simulink model "uas_hoops"  (R2021a)
settings: Solver=FixedStepAuto  StartTime=0.0  StopTime=1  FixedStep=0.04  RelTol=1e-3
model workspace: external: MAT-File (data not in the file)
libraries: robotlib x4
settings Model: EnablePacing=on  OrderedModelArguments=off  Creator=david  LastModifiedBy=david
settings SolverCC: AlgebraicLoopSolver=TrustRegion
settings DataIOCC: LimitDataPoints=on  MaxDataPoints=10000
settings OptimizationCC: EnhancedBackFolding=on  PassReuseOutputArgsThreshold=0  ZeroExternalMemoryAtStartup=off  ZeroInternalMemoryAtStartup=off  MaxStackSize=64  OptimizeBlockOrder=speed  DifferentSizesBufferReuse=on  OptimizationCustomize=off
settings DebuggingCC: ParameterTunabilityLossMsg=error  AllowSymbolicDim=off  SFUnexpectedBacktrackingDiag=warning  SFNoUnconditionalDefaultTransitionDiag=warning  SFExecutionAtInitializationDiag=none  SFMachineParentedDataDiag=warning  UnderSpecifiedDimensionMsg=warning  ArithmeticOperatorsInVariantConditions=warning
settings HardwareCC: ProdBitPerPointer=32  ProdBitPerSizeT=32  ProdBitPerPtrDiffT=32  ProdLargestAtomicFloat=None  ProdIntDivRoundTo=Undefined  ProdEndianess=Unspecified  ProdWordSize=32  ProdHWDeviceType=Generic->Unspecified (assume 32-bit Generic)  UseEmbeddedCoderFeatures=off
settings SFSimCC: SimUseLocalCustomCode=off  MATLABDynamicMemAlloc=off  CustomCodeUndefinedFunction=UseInterfaceOnly  SimTargetLang=C++
settings RTWCC: SystemTargetFile=ert.tlc  HardwareBoard=Robot Operating System (ROS)  TLCOptions="-aInlineSetEventsForThisBaseRateFcn=TLC_FALSE -aSuppressMultiTaskScheduler=TLC_FALSE  -aRateBasedStepFcn=0"  TemplateMakefile=ert_default_tmf  RTWUseLocalCustomCode=off  Toolchain=Catkin  TargetLang=C++
settings CodeAppCC: ForceParamTrailComments=on  OperatorAnnotations=on
settings ERTTargetCC: ERTCustomFileBanners=off  CodeInterfacePackaging=C++ class  SupportContinuousTime=on  SupportNonInlinedSFcns=on  RemoveResetFunc=off  ModelStepFunctionPrototypeControlCompliant=off  RootIOFormat=Structure reference
settings ConfigComp: CovMetricSettings=dw  CovSaveCumulativeToWorkspaceVar=on  CovSaveSingleToWorkspaceVar=on  CovExternalEMLEnable=off  CovSFcnEnable=off
settings SimscapeCC: SimscapeLogType=all  SimscapeLogSimulationStatistics=on  SimscapeLogDataHistory=10000

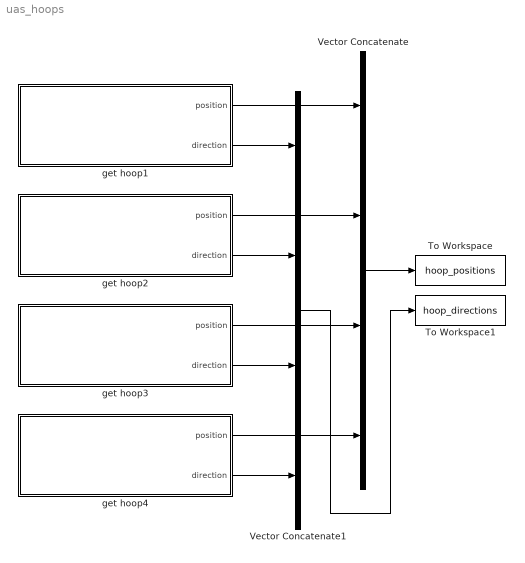
== system uas_hoops ==
  To Workspace : ToWorkspace  VariableName=hoop_positions  SaveFormat=Timeseries  SampleTime=-1
  To Workspace1 : ToWorkspace  VariableName=hoop_directions  SaveFormat=Timeseries  SampleTime=-1
  Vector Concatenate : Concatenate  NumInputs=4  Mode=Multidimensional array  ConcatenateDimension=2
  Vector Concatenate1 : Concatenate  NumInputs=4  Mode=Multidimensional array  ConcatenateDimension=2
  get hoop1 : Subsystem
  get hoop2 : Subsystem
  get hoop3 : Subsystem
  get hoop4 : Subsystem
  wires:
  get hoop1/1(position) -> Vector Concatenate/1
  get hoop2/1(position) -> Vector Concatenate/2
  get hoop3/1(position) -> Vector Concatenate/3
  get hoop4/1(position) -> Vector Concatenate/4
  Vector Concatenate/1 -> To Workspace/1
  Vector Concatenate1/1 -> To Workspace1/1
  get hoop1/2(direction) -> Vector Concatenate1/1
  get hoop2/2(direction) -> Vector Concatenate1/2
  get hoop3/2(direction) -> Vector Concatenate1/3
  get hoop4/2(direction) -> Vector Concatenate1/4

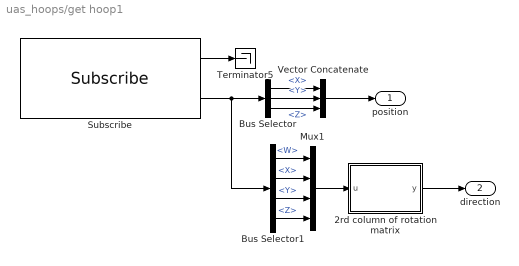
== system uas_hoops/get hoop1 ==
  2rd column of rotation matrix : MATLAB Function  TreatAsAtomicUnit=on
  Bus Selector : BusSelector  OutputSignals=Pose.Position.X,Pose.Position.Y,Pose.Position.Z
  Bus Selector1 : BusSelector  OutputSignals=Pose.Orientation.W,Pose.Orientation.X,Pose.Orientation.Y,Pose.Orientation.Z
  Mux1 : Mux
  Subscribe : robotlib/Subscribe  topicSource=Specify your own  topic=/vrpn_client_node/hoop1/pose  messageType=geometry_msgs/PoseStamped  SampleTime=-1  legacyBusStruct=off  messageQueueLength=1
  Terminator5 : Terminator
  Vector Concatenate : Concatenate  NumInputs=3  Mode=Multidimensional array
  position : Outport
  direction : Outport  Port=2
  wires:
  Subscribe/2 -> Bus Selector1/1, Bus Selector/1
  Bus Selector/3 -> Vector Concatenate/3  "<Z>"
  Bus Selector/1 -> Vector Concatenate/1  "<X>"
  Bus Selector/2 -> Vector Concatenate/2  "<Y>"
  Subscribe/1 -> Terminator5/1
  Bus Selector1/1 -> Mux1/1  "<W>"
  Bus Selector1/2 -> Mux1/2  "<X>"
  Bus Selector1/3 -> Mux1/3  "<Y>"
  Bus Selector1/4 -> Mux1/4  "<Z>"
  Mux1/1 -> 2rd column of rotation matrix/1(u)
  2rd column of rotation matrix/1(y) -> direction/1
  Vector Concatenate/1 -> position/1

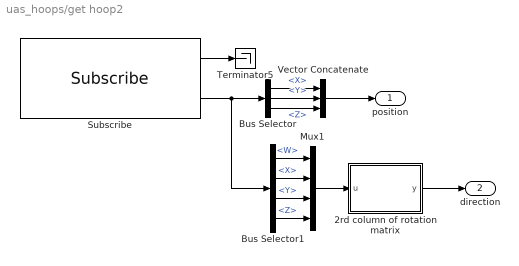
== system uas_hoops/get hoop2 ==
  2rd column of rotation matrix : MATLAB Function  TreatAsAtomicUnit=on
  Bus Selector : BusSelector  OutputSignals=Pose.Position.X,Pose.Position.Y,Pose.Position.Z
  Bus Selector1 : BusSelector  OutputSignals=Pose.Orientation.W,Pose.Orientation.X,Pose.Orientation.Y,Pose.Orientation.Z
  Mux1 : Mux
  Subscribe : robotlib/Subscribe  topicSource=Specify your own  topic=/vrpn_client_node/hoop2/pose  messageType=geometry_msgs/PoseStamped  SampleTime=-1  legacyBusStruct=off  messageQueueLength=1
  Terminator5 : Terminator
  Vector Concatenate : Concatenate  NumInputs=3  Mode=Multidimensional array
  position : Outport
  direction : Outport  Port=2
  wires:
  Subscribe/2 -> Bus Selector1/1, Bus Selector/1
  Bus Selector/3 -> Vector Concatenate/3  "<Z>"
  Bus Selector/1 -> Vector Concatenate/1  "<X>"
  Bus Selector/2 -> Vector Concatenate/2  "<Y>"
  Subscribe/1 -> Terminator5/1
  Bus Selector1/1 -> Mux1/1  "<W>"
  Bus Selector1/2 -> Mux1/2  "<X>"
  Bus Selector1/3 -> Mux1/3  "<Y>"
  Bus Selector1/4 -> Mux1/4  "<Z>"
  Mux1/1 -> 2rd column of rotation matrix/1(u)
  2rd column of rotation matrix/1(y) -> direction/1
  Vector Concatenate/1 -> position/1

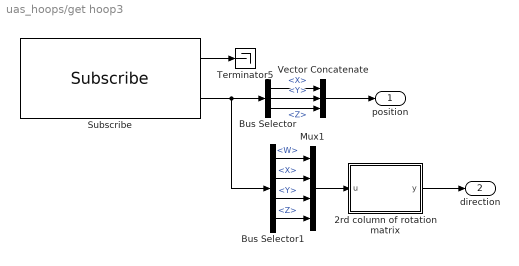
== system uas_hoops/get hoop3 ==
  2rd column of rotation matrix : MATLAB Function  TreatAsAtomicUnit=on
  Bus Selector : BusSelector  OutputSignals=Pose.Position.X,Pose.Position.Y,Pose.Position.Z
  Bus Selector1 : BusSelector  OutputSignals=Pose.Orientation.W,Pose.Orientation.X,Pose.Orientation.Y,Pose.Orientation.Z
  Mux1 : Mux
  Subscribe : robotlib/Subscribe  topicSource=Specify your own  topic=/vrpn_client_node/hoop3/pose  messageType=geometry_msgs/PoseStamped  SampleTime=-1  legacyBusStruct=off  messageQueueLength=1
  Terminator5 : Terminator
  Vector Concatenate : Concatenate  NumInputs=3  Mode=Multidimensional array
  position : Outport
  direction : Outport  Port=2
  wires:
  Subscribe/2 -> Bus Selector1/1, Bus Selector/1
  Bus Selector/3 -> Vector Concatenate/3  "<Z>"
  Bus Selector/1 -> Vector Concatenate/1  "<X>"
  Bus Selector/2 -> Vector Concatenate/2  "<Y>"
  Subscribe/1 -> Terminator5/1
  Bus Selector1/1 -> Mux1/1  "<W>"
  Bus Selector1/2 -> Mux1/2  "<X>"
  Bus Selector1/3 -> Mux1/3  "<Y>"
  Bus Selector1/4 -> Mux1/4  "<Z>"
  Mux1/1 -> 2rd column of rotation matrix/1(u)
  2rd column of rotation matrix/1(y) -> direction/1
  Vector Concatenate/1 -> position/1

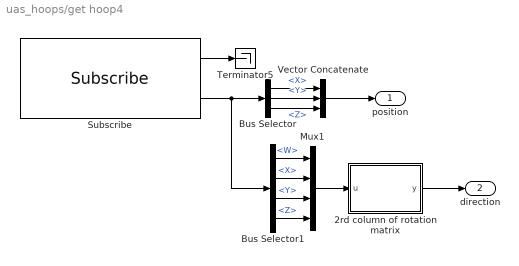
== system uas_hoops/get hoop4 ==
  2rd column of rotation matrix : MATLAB Function  TreatAsAtomicUnit=on
  Bus Selector : BusSelector  OutputSignals=Pose.Position.X,Pose.Position.Y,Pose.Position.Z
  Bus Selector1 : BusSelector  OutputSignals=Pose.Orientation.W,Pose.Orientation.X,Pose.Orientation.Y,Pose.Orientation.Z
  Mux1 : Mux
  Subscribe : robotlib/Subscribe  topicSource=Specify your own  topic=/vrpn_client_node/hoop4/pose  messageType=geometry_msgs/PoseStamped  SampleTime=-1  legacyBusStruct=off  messageQueueLength=1
  Terminator5 : Terminator
  Vector Concatenate : Concatenate  NumInputs=3  Mode=Multidimensional array
  position : Outport
  direction : Outport  Port=2
  wires:
  Subscribe/2 -> Bus Selector1/1, Bus Selector/1
  Bus Selector/3 -> Vector Concatenate/3  "<Z>"
  Bus Selector/1 -> Vector Concatenate/1  "<X>"
  Bus Selector/2 -> Vector Concatenate/2  "<Y>"
  Subscribe/1 -> Terminator5/1
  Bus Selector1/1 -> Mux1/1  "<W>"
  Bus Selector1/2 -> Mux1/2  "<X>"
  Bus Selector1/3 -> Mux1/3  "<Y>"
  Bus Selector1/4 -> Mux1/4  "<Z>"
  Mux1/1 -> 2rd column of rotation matrix/1(u)
  2rd column of rotation matrix/1(y) -> direction/1
  Vector Concatenate/1 -> position/1

== matlab function uas_hoops/get hoop2/2rd column of rotation matrix ==
  data: u input size=[1 4]; y output size=[3 1]
function y = get_r2(u)

R = quat2rotm(u);

y = R(:,2);

== matlab function uas_hoops/get hoop3/2rd column of rotation matrix ==
  data: u input size=[1 4]; y output size=[3 1]
function y = get_r2(u)

R = quat2rotm(u);

y = R(:,2);

== matlab function uas_hoops/get hoop4/2rd column of rotation matrix ==
  data: u input size=[1 4]; y output size=[3 1]
function y = get_r2(u)

R = quat2rotm(u);

y = R(:,2);

== matlab function uas_hoops/get hoop1/2rd column of rotation matrix ==
  data: u input size=[1 4]; y output size=[3 1]
function y = get_r2(u)

R = quat2rotm(u);

y = R(:,2);
